simulink model "PFC_Controller"  (R2021b)
settings: configuration reference "Configuration" (kept outside this file)
settings Model: DataDictionary=ZC_EVPowerSystem.sldd  Creator=ykamatan  LastModifiedBy=ykamatan
settings ConfigSetRef: SourceName=Configuration

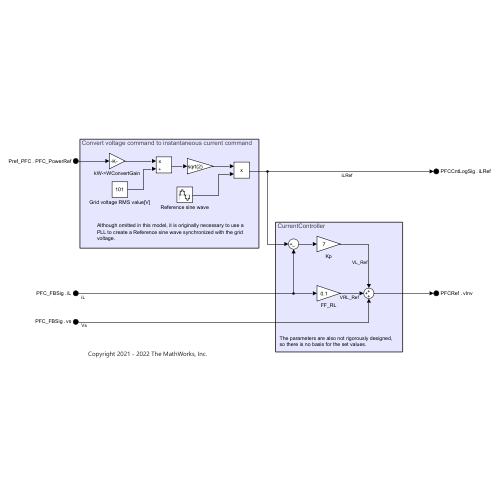
[thumbnail: Simulink's stored preview of the top-level diagram]
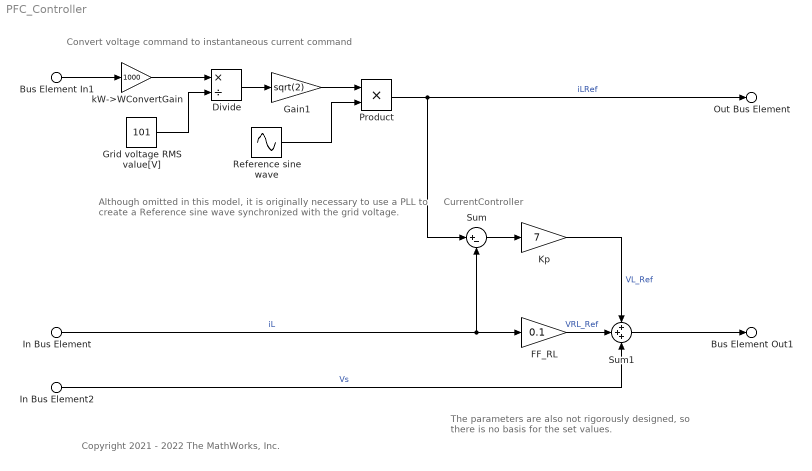
== system PFC_Controller ==
  note: The parameters are also not rigorously designed, so there is no basis for the set values.
  note: Although omitted in this model, it is originally necessary to use a PLL to create a Reference sine wave synchronized with the grid voltage.
  note: CurrentController
  note: Convert voltage command to instantaneous current command
  note: Copyright 2021 - 2022 The MathWorks, Inc.
  Bus Element In1 : Inport  PortName=Pref_PFC  Element=PFC_PowerRef
  In Bus Element2 : Inport  Port=2  PortName=PFC_FBSig  Element=vs
  In Bus Element : Inport  Port=2  PortName=PFC_FBSig  Element=iL
  Divide : Product  Inputs=*/
  FF_RL : Gain  Gain=0.1
  Gain1 : Gain  Gain=sqrt(2)
  Grid voltage RMS value[V] : Constant  Value=101
  Kp : Gain  Gain=7
  Product : Product
  Reference sine wave : Sin  Amplitude=-1  Frequency=2*pi*60  SampleTime=1/10000
  Sum : Sum  Inputs=|+-
  Sum1 : Sum  Inputs=+++
  kW->WConvertGain : Gain  Gain=1000
  Bus Element Out1 : Outport  PortName=PFCRef  Element=vInv
  Out Bus Element : Outport  Port=2  PortName=PFCCntLogSig  Element=iLRef
  wires:
  Sum1/1 -> Bus Element Out1/1
  In Bus Element2/1 -> Sum1/3  "Vs"
  In Bus Element/1 -> Sum/2, FF_RL/1  "iL"
  Product/1 -> Sum/1, Out Bus Element/1  "iLRef"
  Reference sine wave/1 -> Product/2
  Bus Element In1/1 -> kW->WConvertGain/1
  Gain1/1 -> Product/1
  Divide/1 -> Gain1/1
  Grid voltage RMS value[V]/1 -> Divide/2
  kW->WConvertGain/1 -> Divide/1
  Kp/1 -> Sum1/1  "VL_Ref"
  Sum/1 -> Kp/1
  FF_RL/1 -> Sum1/2  "VRL_Ref"
